simulink model "x13_foc_pll"  (R2023b)
settings: Solver=VariableStepAuto  StartTime=0.0  StopTime=0.5  RelTol=1e-3
values from neighbouring files (symbols this model uses):
  pll_ki = pll_wn*pll_wn    (= 98696.0440109)    [foc_para.m]
  pll_kp = 2*pll_wn    (= 628.318530718)    [foc_para.m]
  pll_out_max = 333*2*pi*2    (= 4184.60141458)    [foc_para.m]
  Ts = 1/SwitchFrequency    (= 5e-05)    [foc_para.m]
undefined symbols (not defined in the file or in its folder): DiscIntNeverNeededParam
libraries: spspowerguiLib x1
settings Model: Creator=disnox  LastModifiedBy=disno
settings DataIOCC: ReturnWorkspaceOutputs=off
settings DebuggingCC: ParameterPrecisionLossMsg=none

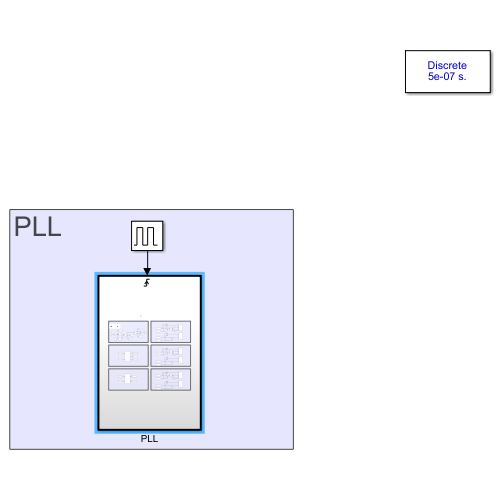
[thumbnail: Simulink's stored preview of the top-level diagram]
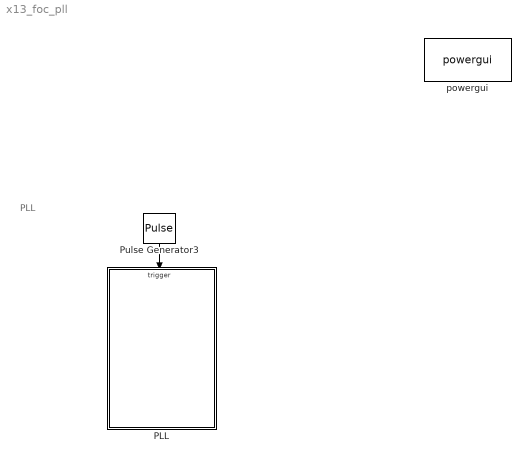
== system x13_foc_pll ==
  note: PLL
  PLL : Subsystem
  Pulse Generator3 : DiscretePulseGenerator  PulseType=Time based  Period=Ts  PulseWidth=50
  powergui : spspowerguiLib/powergui  SimulationMode=Discrete  SampleTime=Ts/100  frequency=60  Iterations=50  frequencyindice=0  Pbase=100e6  ErrMax=1e-4  UnitsV=kV  UnitsW=MW  buscounter=0  FunctionMessages=off  echomessages=off  EnableUseOfTLC=off  CurrentSourceSwitches=off  DisableSnubberDevices=off  DisableRonSwitches=off  DisableVfSwitches=off  DisplayEquations=off  AutomaticDiscreteSolvers=off  SolverType=Tustin/Backward Euler (TBE)  Interpol=off  ExternalGateDelay=off  methode=off  Ts=0  x0status=blocks  SPID=off  SwTol=0  HookPort=off  NonlinearTolerance=1e-4  nMaxIteration=100  ContinueOnMaxIteration=off  RestoreLinks=warning  ResistiveCurrentMeasurement=off  Frange=[0:2:500]  Ylog=off  Xlog=on  ShowGrid=off  save=off  variable=ZData  structure=0  ZoomFFT=off  StartTime=0.0  cycles=1  DisplayStyle=1  fundamental=60  FreqAxis=off  MaxFrequency=1000  frequencyindicesteady=1  RmsSteady=1  display=off
  wires:
  Pulse Generator3/1 -> PLL/Trigger

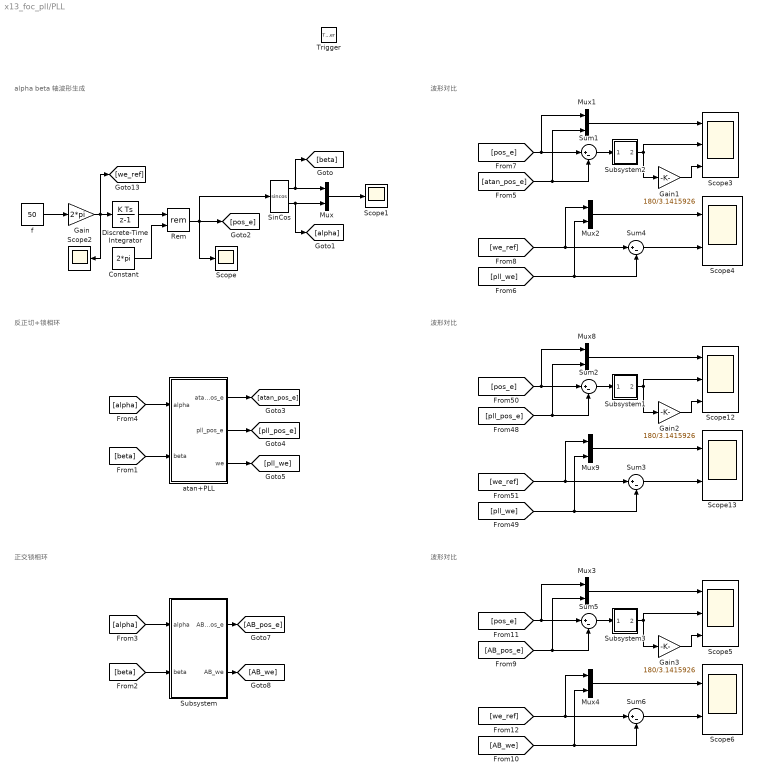
== system x13_foc_pll/PLL ==
  note: 反正切+锁相环
  note: alpha beta 轴波形生成
  note: 正交锁相环
  note: 波形对比
  note: 波形对比
  note: 波形对比
  Trigger : TriggerPort  VariantControl=(inherit)
  Constant : Constant  Value=2*pi
  Discrete-Time Integrator : DiscreteIntegrator  SampleTime=-1  ICPrevOutput=DiscIntNeverNeededParam  ICPrevScaledInput=DiscIntNeverNeededParam
  Gain : Gain  Gain=2*pi
  Gain1 : Gain  Gain=180/3.1415926
  Gain2 : Gain  Gain=180/3.1415926
  Gain3 : Gain  Gain=180/3.1415926
  Mux{,1..4,8..9} (7 alike) : Mux  Inputs=2
  Rem : Math  Operator=rem
  Scope : Scope
  Scope1 : Scope
  Scope12 : Scope  NumInputPorts=3
  Scope13 : Scope  NumInputPorts=2
  Scope2 : Scope
  Scope3 : Scope  NumInputPorts=3
  Scope4 : Scope  NumInputPorts=2
  Scope5 : Scope  NumInputPorts=3
  Scope6 : Scope  NumInputPorts=2
  SinCos : Trigonometry  Operator=sincos
  Subsystem : Subsystem  mask{gain=1, pll_kp=pll_kp, pll_ki=pll_ki, pll_out_max=pll_out_max}
      mask DialogControl ParameterGroupVar Prompt: 参数
      mask Display: disp('AB_PLL')
  Subsystem1 : Subsystem
      mask DialogControl ParameterGroupVar Prompt: 参数
      mask Display: disp('0-2pi')
  Subsystem2 : Subsystem
      mask DialogControl ParameterGroupVar Prompt: 参数
      mask Display: disp('0-2pi')
  Subsystem3 : Subsystem
      mask DialogControl ParameterGroupVar Prompt: 参数
      mask Display: disp('0-2pi')
  Sum{1..6} (6 alike) : Sum  Inputs=|+-
  atan+PLL : Subsystem  mask{pll_kp=pll_kp, pll_ki=pll_ki, pll_out_max=pll_out_max}
      mask DialogControl ParameterGroupVar Prompt: 参数
      mask Display: disp('PLL')
  f : Constant  Value=50
  wires:
  SinCos/2 -> [alpha], Mux/2
  f/1 -> Gain/1
  Rem/1 -> [pos_e], SinCos/1, Scope/1
  Discrete-Time Integrator/1 -> Rem/1
  SinCos/1 -> [beta], Mux/1
  Gain/1 -> Discrete-Time Integrator/1, Scope2/1, [we_ref]
  Constant/1 -> Rem/2
  Mux/1 -> Scope1/1
  atan+PLL/1(atan_pos_e) -> [atan_pos_e]
  atan+PLL/2(pll_pos_e) -> [pll_pos_e]
  atan+PLL/3(we) -> [pll_we]
  [alpha] -> atan+PLL/1(alpha)
  [beta] -> atan+PLL/2(beta)
  Subsystem/1(AB_pos_e) -> [AB_pos_e]
  Subsystem/2(AB_we) -> [AB_we]
  [pll_we] -> Sum3/2, Mux9/2
  Mux8/1 -> Scope12/1
  Sum2/1 -> Subsystem1/1("1 ")
  [pos_e] -> Mux8/1, Sum2/1
  Gain2/1 -> Scope12/3
  [pll_pos_e] -> Sum2/2, Mux8/2
  Mux9/1 -> Scope13/1
  [we_ref] -> Sum3/1, Mux9/1
  Sum3/1 -> Scope13/2
  Subsystem1/1(2) -> Scope12/2, Gain2/1
  Sum4/1 -> Scope4/2
  Mux2/1 -> Scope4/1
  [pos_e] -> Mux1/1, Sum1/1
  Sum1/1 -> Subsystem2/1("1 ")
  [pll_we] -> Sum4/2, Mux2/2
  [atan_pos_e] -> Sum1/2, Mux1/2
  Gain1/1 -> Scope3/3
  Mux1/1 -> Scope3/1
  [we_ref] -> Sum4/1, Mux2/1
  Subsystem2/1(2) -> Scope3/2, Gain1/1
  Sum6/1 -> Scope6/2
  Mux4/1 -> Scope6/1
  [pos_e] -> Mux3/1, Sum5/1
  Sum5/1 -> Subsystem3/1("1 ")
  [AB_we] -> Sum6/2, Mux4/2
  [AB_pos_e] -> Sum5/2, Mux3/2
  Gain3/1 -> Scope5/3
  Mux3/1 -> Scope5/1
  [we_ref] -> Sum6/1, Mux4/1
  Subsystem3/1(2) -> Scope5/2, Gain3/1
  [alpha] -> Subsystem/1(alpha)
  [beta] -> Subsystem/2(beta)

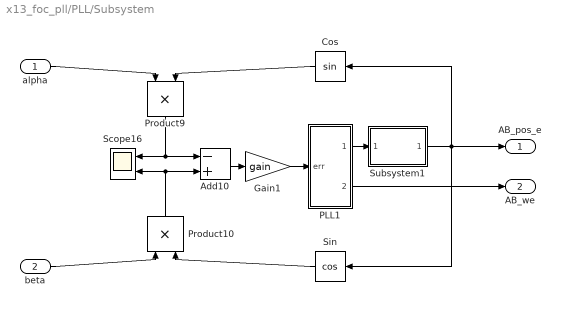
== system x13_foc_pll/PLL/Subsystem ==
  alpha : Inport
  beta : Inport  Port=2
  Add10 : Sum  Inputs=-+
  Cos : Trigonometry
  Gain1 : Gain  Gain=gain
  PLL1 : Subsystem  TreatAsAtomicUnit=on
      settings: RTWSystemCode=Nonreusable function  RTWFcnNameOpts=Use subsystem name
  Product10 : Product
  Product9 : Product
  Scope16 : Scope  NumInputPorts=2
  Sin : Trigonometry  Operator=cos
  Subsystem1 : Subsystem
  AB_pos_e : Outport
  AB_we : Outport  Port=2
  wires:
  PLL1/1(angle) -> Subsystem1/1(angle)
  Product10/1 -> Add10/2, Scope16/2
  Product9/1 -> Scope16/1, Add10/1
  PLL1/2(speed) -> AB_we/1
  Cos/1 -> Product9/2
  Subsystem1/1(theta) -> Cos/1, Sin/1, AB_pos_e/1
  Sin/1 -> Product10/2
  beta/1 -> Product10/1
  Gain1/1 -> PLL1/1(err)
  Add10/1 -> Gain1/1
  alpha/1 -> Product9/1

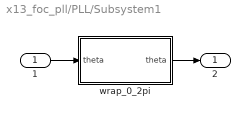
== system x13_foc_pll/PLL/Subsystem1 ==
  "1 " : Inport
  wrap_0_2pi : MATLAB Function  TreatAsAtomicUnit=on
  2 : Outport
  wires:
  "1 "/1 -> wrap_0_2pi/1("theta ")
  wrap_0_2pi/1(theta) -> 2/1

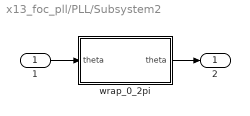
== system x13_foc_pll/PLL/Subsystem2 ==
  "1 " : Inport
  wrap_0_2pi : MATLAB Function  TreatAsAtomicUnit=on
  2 : Outport
  wires:
  "1 "/1 -> wrap_0_2pi/1("theta ")
  wrap_0_2pi/1(theta) -> 2/1

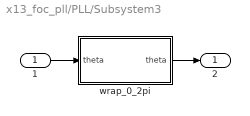
== system x13_foc_pll/PLL/Subsystem3 ==
  "1 " : Inport
  wrap_0_2pi : MATLAB Function  TreatAsAtomicUnit=on
  2 : Outport
  wires:
  "1 "/1 -> wrap_0_2pi/1("theta ")
  wrap_0_2pi/1(theta) -> 2/1

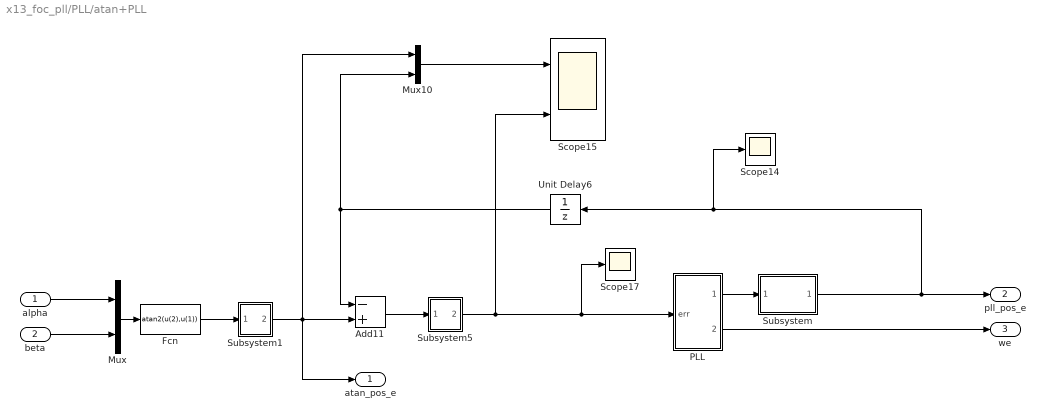
== system x13_foc_pll/PLL/atan+PLL ==
  alpha : Inport
  beta : Inport  Port=2
  Add11 : Sum  Inputs=-+
  Fcn : Fcn  Expr=atan2(u(2),u(1))
  Mux : Mux  Inputs=2
  Mux10 : Mux  Inputs=2
  PLL : Subsystem  TreatAsAtomicUnit=on
      settings: RTWSystemCode=Nonreusable function  RTWFcnNameOpts=Use subsystem name
  Scope14 : Scope
  Scope15 : Scope  NumInputPorts=2
  Scope17 : Scope
  Subsystem : Subsystem
  Subsystem1 : Subsystem
      mask DialogControl ParameterGroupVar Prompt: 参数
      mask Display: disp('0-2pi')
  Subsystem5 : Subsystem
      mask DialogControl ParameterGroupVar Prompt: 参数
      mask Display: disp('-pi-pi')
  Unit Delay6 : UnitDelay  SampleTime=-1  HasFrameUpgradeWarning=on
  atan_pos_e : Outport
  pll_pos_e : Outport  Port=2
  we : Outport  Port=3
  wires:
  Unit Delay6/1 -> Mux10/2, Add11/1
  Fcn/1 -> Subsystem1/1("1 ")
  Add11/1 -> Subsystem5/1("1 ")
  Subsystem1/1(2) -> atan_pos_e/1, Mux10/1, Add11/2
  Subsystem5/1(2) -> Scope15/2, Scope17/1, PLL/1(err)
  Subsystem/1(theta) -> pll_pos_e/1, Scope14/1, Unit Delay6/1
  PLL/1(angle) -> Subsystem/1(angle)
  Mux10/1 -> Scope15/1
  PLL/2(speed) -> we/1
  Mux/1 -> Fcn/1
  alpha/1 -> Mux/1
  beta/1 -> Mux/2

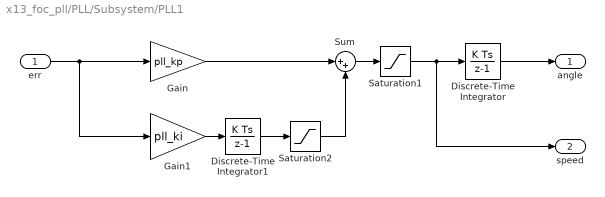
== system x13_foc_pll/PLL/Subsystem/PLL1 ==
  err : Inport
  Discrete-Time Integrator : DiscreteIntegrator  SampleTime=-1  ICPrevOutput=DiscIntNeverNeededParam  ICPrevScaledInput=DiscIntNeverNeededParam
  Discrete-Time Integrator1 : DiscreteIntegrator  SampleTime=-1  ICPrevOutput=DiscIntNeverNeededParam  ICPrevScaledInput=DiscIntNeverNeededParam
  Gain : Gain  Gain=pll_kp
  Gain1 : Gain  Gain=pll_ki
  Saturation1 : Saturate  UpperLimit=pll_out_max  LowerLimit=-pll_out_max
  Saturation2 : Saturate  UpperLimit=pll_out_max  LowerLimit=-pll_out_max
  Sum : Sum  Inputs=|++
  angle : Outport
  speed : Outport  Port=2
  wires:
  err/1 -> Gain1/1, Gain/1
  Gain/1 -> Sum/1
  Gain1/1 -> Discrete-Time Integrator1/1
  Discrete-Time Integrator1/1 -> Saturation2/1
  Saturation2/1 -> Sum/2
  Sum/1 -> Saturation1/1
  Saturation1/1 -> speed/1, Discrete-Time Integrator/1
  Discrete-Time Integrator/1 -> angle/1

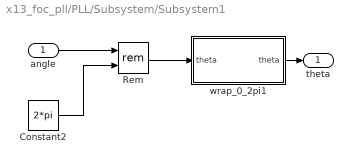
== system x13_foc_pll/PLL/Subsystem/Subsystem1 ==
  angle : Inport
  Constant2 : Constant  Value=2*pi
  Rem : Math  Operator=rem
  wrap_0_2pi1 : MATLAB Function  TreatAsAtomicUnit=on
  theta : Outport
  wires:
  wrap_0_2pi1/1(theta) -> theta/1
  Constant2/1 -> Rem/2
  Rem/1 -> wrap_0_2pi1/1("theta ")
  angle/1 -> Rem/1

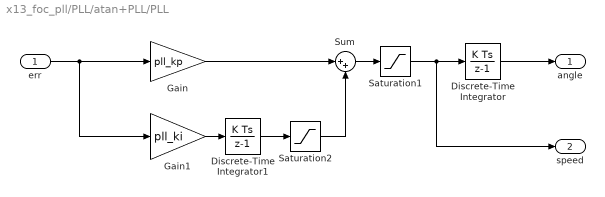
== system x13_foc_pll/PLL/atan+PLL/PLL ==
  err : Inport
  Discrete-Time Integrator : DiscreteIntegrator  SampleTime=-1  ICPrevOutput=DiscIntNeverNeededParam  ICPrevScaledInput=DiscIntNeverNeededParam
  Discrete-Time Integrator1 : DiscreteIntegrator  SampleTime=-1  ICPrevOutput=DiscIntNeverNeededParam  ICPrevScaledInput=DiscIntNeverNeededParam
  Gain : Gain  Gain=pll_kp
  Gain1 : Gain  Gain=pll_ki
  Saturation1 : Saturate  UpperLimit=pll_out_max  LowerLimit=-pll_out_max
  Saturation2 : Saturate  UpperLimit=pll_out_max  LowerLimit=-pll_out_max
  Sum : Sum  Inputs=|++
  angle : Outport
  speed : Outport  Port=2
  wires:
  err/1 -> Gain1/1, Gain/1
  Gain/1 -> Sum/1
  Gain1/1 -> Discrete-Time Integrator1/1
  Discrete-Time Integrator1/1 -> Saturation2/1
  Saturation2/1 -> Sum/2
  Sum/1 -> Saturation1/1
  Saturation1/1 -> speed/1, Discrete-Time Integrator/1
  Discrete-Time Integrator/1 -> angle/1

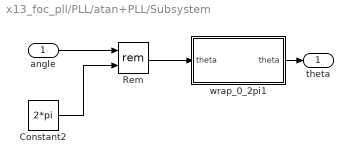
== system x13_foc_pll/PLL/atan+PLL/Subsystem ==
  angle : Inport
  Constant2 : Constant  Value=2*pi
  Rem : Math  Operator=rem
  wrap_0_2pi1 : MATLAB Function  TreatAsAtomicUnit=on
  theta : Outport
  wires:
  wrap_0_2pi1/1(theta) -> theta/1
  Constant2/1 -> Rem/2
  Rem/1 -> wrap_0_2pi1/1("theta ")
  angle/1 -> Rem/1

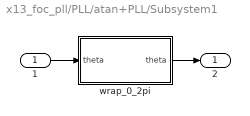
== system x13_foc_pll/PLL/atan+PLL/Subsystem1 ==
  "1 " : Inport
  wrap_0_2pi : MATLAB Function  TreatAsAtomicUnit=on
  2 : Outport
  wires:
  "1 "/1 -> wrap_0_2pi/1("theta ")
  wrap_0_2pi/1(theta) -> 2/1

== system x13_foc_pll/PLL/atan+PLL/Subsystem5 ==
  "1 " : Inport
  wrap_pm_pi1 : MATLAB Function  TreatAsAtomicUnit=on
  2 : Outport
  wires:
  "1 "/1 -> wrap_pm_pi1/1("theta ")
  wrap_pm_pi1/1(theta) -> 2/1

== matlab function x13_foc_pll/PLL/Subsystem2/wrap_0_2pi ==
  data: theta output; theta input
function theta = wrap_0_2pi(theta)

    M_2PI = 2*pi;
    
    if theta > M_2PI
        theta = theta - M_2PI;
    elseif theta < 0
        theta = theta + M_2PI;
    end
end

== matlab function x13_foc_pll/PLL/Subsystem1/wrap_0_2pi ==
  data: theta output; theta input
function theta = wrap_0_2pi(theta)

    M_2PI = 2*pi;
    
    if theta > M_2PI
        theta = theta - M_2PI;
    elseif theta < 0
        theta = theta + M_2PI;
    end
end

== matlab function x13_foc_pll/PLL/Subsystem3/wrap_0_2pi ==
  data: theta output; theta input
function theta = wrap_0_2pi(theta)

    M_2PI = 2*pi;
    
    if theta > M_2PI
        theta = theta - M_2PI;
    elseif theta < 0
        theta = theta + M_2PI;
    end
end

== matlab function x13_foc_pll/PLL/Subsystem/Subsystem1/wrap_0_2pi1 ==
  data: theta output; theta input
function theta = wrap_0_2pi(theta)

    M_2PI = 2*pi;
    
    if theta > M_2PI
        theta = theta - M_2PI;
    elseif theta < 0
        theta = theta + M_2PI;
    end
end

== matlab function x13_foc_pll/PLL/atan+PLL/Subsystem1/wrap_0_2pi ==
  data: theta output; theta input
function theta = wrap_0_2pi(theta)

    M_2PI = 2*pi;
    
    if theta > M_2PI
        theta = theta - M_2PI;
    elseif theta < 0
        theta = theta + M_2PI;
    end
end

== matlab function x13_foc_pll/PLL/atan+PLL/Subsystem/wrap_0_2pi1 ==
  data: theta output; theta input
function theta = wrap_0_2pi(theta)

    M_2PI = 2*pi;
    
    if theta > M_2PI
        theta = theta - M_2PI;
    elseif theta < 0
        theta = theta + M_2PI;
    end
end

== matlab function x13_foc_pll/PLL/atan+PLL/Subsystem5/wrap_pm_pi1 ==
  data: theta output; theta input
function theta = wrap_pm_pi(theta)

    M_PI = pi;
    M_2PI = 2*pi;
    
    if theta > M_PI
        theta = theta - M_2PI;
    elseif theta < -M_PI
        theta = theta + M_2PI;
    end
end
